simulink model "Control_Allocation_VV"  (R2020b)
settings: Solver=VariableStepAuto  StartTime=0.0  StopTime=10.0  RelTol=1e-3
settings Model: Creator=Jonathan van Zyl  LastModifiedBy=Jonathan van Zyl

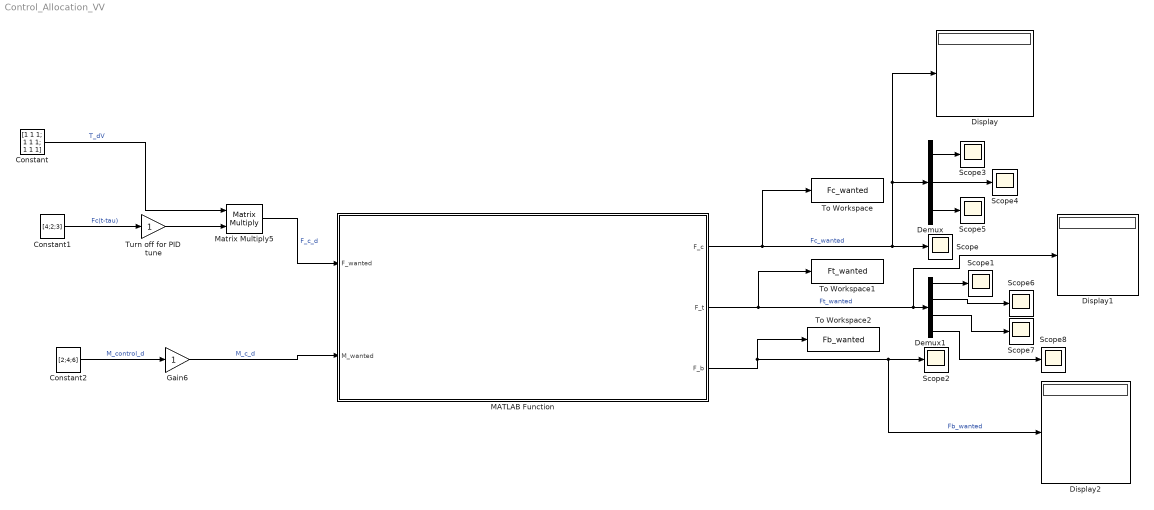
== system Control_Allocation_VV ==
  Constant : Constant  Value=[1 1 1; 1 1 1; 1 1 1]
  Constant1 : Constant  Value=[4;2;3]
  Constant2 : Constant  Value=[2;4;6]
  Demux : Demux  Outputs=3
  Demux1 : Demux
  Display : Display
  Display1 : Display
  Display2 : Display
  Gain6 : Gain
  MATLAB Function : MATLAB Function  TreatAsAtomicUnit=on
  Matrix Multiply5 : Product  Multiplication=Matrix(*)
  Scope{,1..8} (9 alike) : Scope
  To Workspace : ToWorkspace  VariableName=Fc_wanted  SaveFormat=Timeseries  SampleTime=-1
  To Workspace1 : ToWorkspace  VariableName=Ft_wanted  SaveFormat=Timeseries  SampleTime=-1
  To Workspace2 : ToWorkspace  VariableName=Fb_wanted  SaveFormat=Timeseries  SampleTime=-1
  Turn off for PID tune : Gain
  wires:
  Turn off for PID tune/1 -> Matrix Multiply5/2
  Constant/1 -> Matrix Multiply5/1  "T_dV"
  MATLAB Function/3(F_b) -> Display2/1, Scope2/1, To Workspace2/1  "Fb_wanted"
  Matrix Multiply5/1 -> MATLAB Function/1(F_wanted)  "F_c_d"
  MATLAB Function/1(F_c) -> Display/1, Demux/1, Scope/1, To Workspace/1  "Fc_wanted"
  Gain6/1 -> MATLAB Function/2(M_wanted)  "M_c_d"
  Constant1/1 -> Turn off for PID tune/1  "Fc(t-tau)"
  MATLAB Function/2(F_t) -> Display1/1, Demux1/1, To Workspace1/1  "Ft_wanted"
  Constant2/1 -> Gain6/1  "M_control_d"
  Demux/1 -> Scope3/1
  Demux/2 -> Scope4/1
  Demux/3 -> Scope5/1
  Demux1/1 -> Scope1/1
  Demux1/2 -> Scope6/1
  Demux1/3 -> Scope7/1
  Demux1/4 -> Scope8/1

== matlab function Control_Allocation_VV/MATLAB Function ==
  data: F_wanted input; F_c output; M_wanted input; F_t output; F_b output
function [F_c, F_t, F_b] = propeller_required_forces_control(F_wanted, M_wanted)

%% Load propeller arms data
xc_1 = 0.1;
yc_1 = 0.05;
zc_1 = -0.3;
xc_2 = 0.1;
yc_2 = -0.2;
zc_2 = 0.3;
xc_3 = 0.1;
yc_3 = -0.2;
zc_3 = 0.3;

xt_1 = 0;
yt_1 = -0.9;
zt_1 = 2.4;
xt_2 = 0;
yt_2 = -0.9;
zt_2 = 1.8;
xt_3 = 0;
yt_3 = -0.9;
zt_3 = -1.2;
xt_4 = 0;
yt_4 = -0.9;
zt_4 = -1.2;

xb_1 = -0.01;
yb_1 = 0;
zb_1 = 1.4;
xb_2 = -0.01;
yb_2 = 0;
zb_2 = 1.4;
%xb_3 = -0.01;
%yb_3 = 0;
%zb_3 = 1.4;
%xb_4 = -0.01;
%yb_4 = 0;
%zb_4 = 1.4;
xb_5 = -0.01;
yb_5 = 0;
zb_5 = 1.4;
xb_6 = -0.01;
yb_6 = 0;
zb_6 = 1.4;
%% Decompose force and moment input

F_x = F_wanted(1);
F_y = F_wanted(2);
F_z = F_wanted(3);

M_x = M_wanted(1);
M_y = M_wanted(2);
M_z = M_wanted(3);

%% Find control forces

F_c3 = 2*(M_x + M_y + F_y)/(-yc_1 + zc_1 - yc_2 + zc_2 - 2*yc_3 + 2*zc_3);
F_c2 = F_c3/2;
F_c1 = F_c2;

%% Find top and bottom forces

F_t1 = 1/8 * F_z + M_y/6*(xt_1 + xt_2 + xt_3 + xt_4 + xb_1 + xb_2 + xb_5 + xb_6);
F_t2 = F_t1;
F_t3 = F_t1;
F_t4 = F_t1;
F_b1 = F_t1;
F_b2 = F_t1;
F_b5 = F_t1;
F_b6 = F_t1;

%F_b3 = 1/10 * F_z;
%F_b4 = F_b3;


%% Make matrix
F_c = [F_c1; F_c2; F_c3];
F_t = [F_t1; F_t2; F_t3; F_t4];
F_b = [F_b1; F_b2; F_b5; F_b6];

end
